simulink subsystem "quat2EulerAngles"  (R2026a)
settings: Solver=VariableStepAuto
values from neighbouring files (symbols this model uses):
  navControl = 1    [navParams.sldd]
libraries: aerolibutil x1
settings Model: Creator=maxhu  LastModifiedBy=maxhu

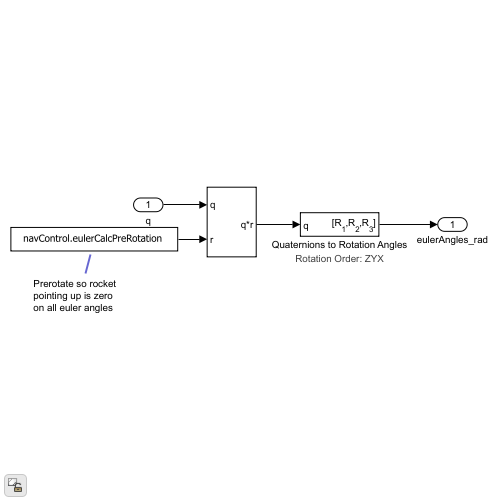
[thumbnail: Simulink's stored preview of the top-level diagram]
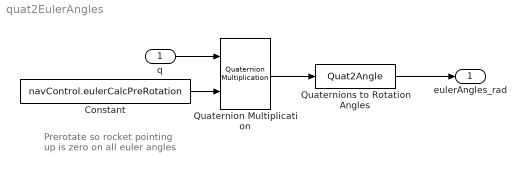
== system quat2EulerAngles ==
  note: Prerotate so rocket pointing up is zero on all euler angles
  q : Inport
  Constant : Constant  Value=navControl.eulerCalcPreRotation
  Quaternion Multiplication : aerolibutil/Quaternion Multiplication
  Quaternions to Rotation Angles : Quat2Angle
      settings: AttributesFormatString=Rotation Order: %<rotationOrder>
  eulerAngles_rad : Outport
  wires:
  Constant/1 -> Quaternion Multiplication/2
  Quaternion Multiplication/1 -> Quaternions to Rotation Angles/1
  q/1 -> Quaternion Multiplication/1
  Quaternions to Rotation Angles/1 -> eulerAngles_rad/1
